simulink subsystem "rocket_rough"  (R2020b)
settings: Solver=VariableStepAuto  StartTime=0.0  StopTime=10.0  RelTol=1e-3
settings Model: Creator=Lucas  LastModifiedBy=Lucas

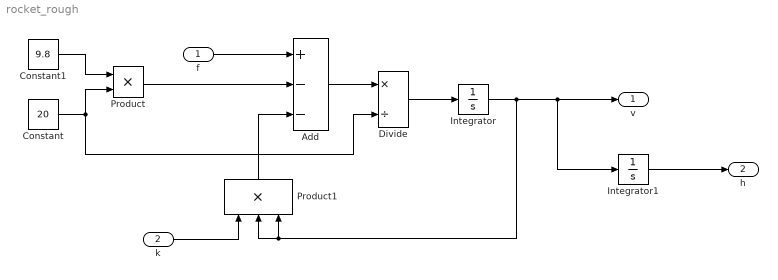
== system rocket_rough ==
  f : Inport
  k : Inport  Port=2
  Add : Sum  Inputs=+--
  Constant : Constant  Value=20
  Constant1 : Constant  Value=9.8
  Divide : Product  Inputs=*/
  Integrator : Integrator
  Integrator1 : Integrator
  Product : Product
  Product1 : Product  Inputs=3
  v : Outport
  h : Outport  Port=2
  wires:
  f/1 -> Add/1
  Product/1 -> Add/2
  Constant/1 -> Product/2, Divide/2
  Constant1/1 -> Product/1
  Product1/1 -> Add/3
  Integrator/1 -> Product1/3, Product1/2, v/1, Integrator1/1
  k/1 -> Product1/1
  Add/1 -> Divide/1
  Divide/1 -> Integrator/1
  Integrator1/1 -> h/1
